simulink model "best_b"  (R2025b)
settings: Solver=FixedStepAuto  StartTime=0.0  StopTime=100  FixedStep=0.1  RelTol=1e-3
undefined symbols (not defined in the file): max_b_dec
libraries: simulink x1
settings Model: Creator=mikol  LastModifiedBy=mikol

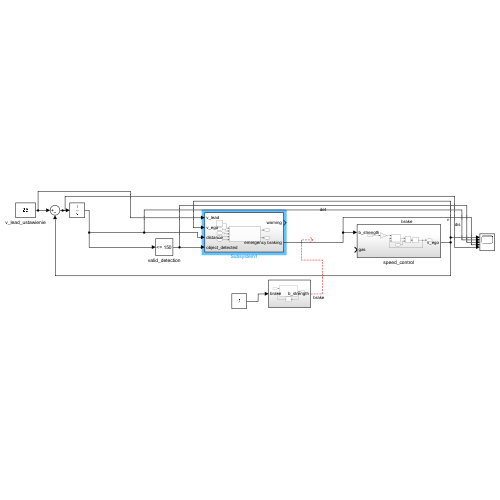
[thumbnail: Simulink's stored preview of the top-level diagram]
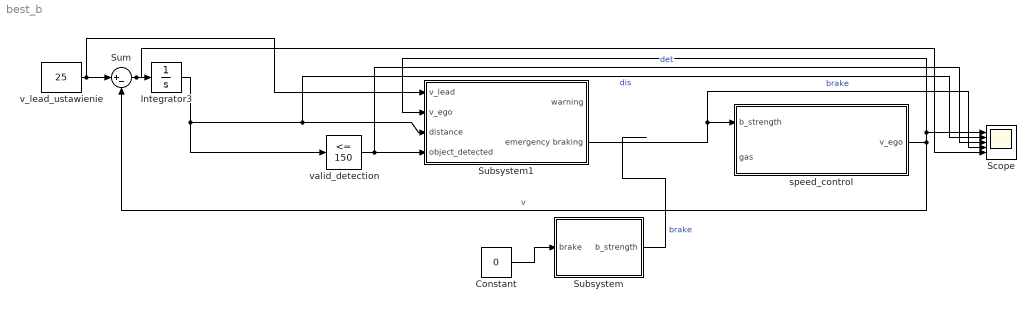
== system best_b ==
  Constant : Constant  Value=0
  Integrator3 : Integrator  InitialCondition=300
  Scope : Scope  NumInputPorts=5
      settings: ActiveDisplayYMinimum=40  ActiveDisplayYMaximum=60
  Subsystem : Subsystem
  Subsystem1 : Subsystem
  Sum : Sum  Inputs=|+-
  speed_control : Subsystem
  v_lead_ustawienie : Constant  Value=25
  valid_detection : simulink/Logic and Bit Operations/Compare To Constant  relop=<=  const=150  OutDataTypeStr=boolean
  wires:
  v_lead_ustawienie/1 -> Subsystem1/1(v_lead), Sum/1
  speed_control/1(v_ego) -> Subsystem1/2(v_ego), Scope/1, Sum/2  "v"
  Integrator3/1 -> Scope/2, Subsystem1/3(distance), valid_detection/1  "dis"
  valid_detection/1 -> Subsystem1/4(object_detected), Scope/3  "det"
  Subsystem/1(b_strength) -> ?  "brake"
  Subsystem1/2(emergency braking) -> Scope/4, speed_control/1(b_strength)  "brake"
  Constant/1 -> Subsystem/1(brake)
  Sum/1 -> Scope/5, Integrator3/1

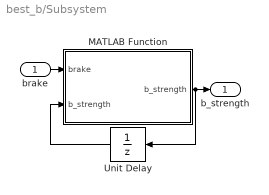
== system best_b/Subsystem ==
  brake : Inport
  MATLAB Function : MATLAB Function  TreatAsAtomicUnit=on
  Unit Delay : UnitDelay  SampleTime=-1  HasFrameUpgradeWarning=on
  b_strength : Outport
  wires:
  brake/1 -> MATLAB Function/1(brake)
  MATLAB Function/1(b_strength) -> b_strength/1, Unit Delay/1
  Unit Delay/1 -> MATLAB Function/2("b_strength ")

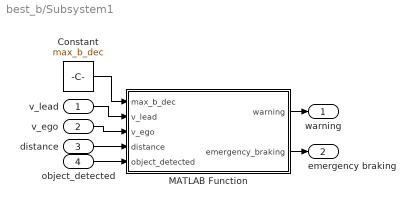
== system best_b/Subsystem1 ==
  v_lead : Inport
  v_ego : Inport  Port=2
  distance : Inport  Port=3
  object_detected : Inport  Port=4
  Constant : Constant  Value=max_b_dec
  MATLAB Function : MATLAB Function  TreatAsAtomicUnit=on
  warning : Outport
  emergency braking : Outport  Port=2
  wires:
  v_ego/1 -> MATLAB Function/3(v_ego)
  MATLAB Function/1(warning) -> warning/1
  v_lead/1 -> MATLAB Function/2(v_lead)
  object_detected/1 -> MATLAB Function/5(object_detected)
  distance/1 -> MATLAB Function/4(distance)
  MATLAB Function/2(emergency_braking) -> emergency braking/1
  Constant/1 -> MATLAB Function/1(max_b_dec)

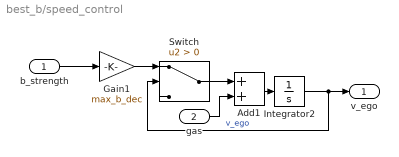
== system best_b/speed_control ==
  b_strength : Inport
  gas : Inport  Port=2
  Add1 : Sum
  Gain1 : Gain  Gain=max_b_dec
  Integrator2 : Integrator  InitialCondition=50
  Switch : Switch  Criteria=u2 > Threshold  SaturateOnIntegerOverflow=off  InputSameDT=off
  v_ego : Outport
  wires:
  Switch/1 -> Add1/1
  Add1/1 -> Integrator2/1
  gas/1 -> Add1/2
  Integrator2/1 -> v_ego/1, Switch/2  "v_ego"
  b_strength/1 -> Gain1/1
  Gain1/1 -> Switch/1

== matlab function best_b/Subsystem1/MATLAB Function ==
  data: max_b_dec input; v_lead input; warning output; v_ego input; distance input; object_detected input; emergency_braking output
function [warning,emergency_braking] = AutonomousEmergencyBraking(max_b_dec,v_lead,v_ego,distance,object_detected)
    if object_detected == false
        warning = 0;
        emergency_braking = 0;
        cant_go_forward = 0;
        return
    end

    braking_distance = distance - v_lead * 0.3;
    v_rel = v_ego - v_lead;
    if v_rel <= 0
        TTR = inf;
        TTres = inf;
    else
        TTR = braking_distance / v_rel;
        TTres = v_rel/max_b_dec;
    end
    FinTres = TTres + 3;
    
    if TTR < FinTres
        warning = 1;
        emergency_braking = 1;
    else
        if TTR < (FinTres + 1.0) && TTR >= FinTres
            warning = 1;
            emergency_braking = 0;
        else
            warning = 0;
            emergency_braking = 0;
        end
    end

== matlab function best_b/Subsystem/MATLAB Function ==
  data: brake input; b_strength input; b_strength output
function b_strength = soft_brake_system(brake,b_strength)
if brake    
    b_strength = b_strength + 0.05 * (1 - b_strength);
else
    b_strength = 0;
end
